simulink model "Supplementary_With_Disturbance"  (R2021a)
settings: Solver=ode4  StartTime=0.0  StopTime=30  FixedStep=0.01  RelTol=1e-3
PreLoadFcn:
  | A = [0	0.0203624760000000	0	0.253756485000000	0.195821163000000	-0.307147013000000	-0.0457249160000000	0	0.0294026210000000	0.282175234000000	0.145131294000000	-0.0517606740000000	0	-0.258258700000000	0.490455158000000	0.458982556000000	0.0397603470000000	0	0.458426005000000	-0.0485128840000000	0.0524025740000000	0.0287956120000000	0	0.0214875670000000	-0.232823046000000	-0.176253649000000	0.0308811180000000	0	-0.0210369990000000	-0.539800040000000	-0.0269942570000000
  | 0.0100000000000000	0.0199027140000000	0	0.254037792000000	0.198666794000000	-0.305673952000000	-0.0462416170000000	0	0.0268056150000000	0.287100361000000	0.149777099000000	-0.0521572690000000	0	-0.262654608000000	0.499529879000000	0.479520423000000	0.0400502210000000	0	0.458640154000000	-0.0508710880000000	0.0506368890000000	0.0290848310000000	0	0.0212556020000000	-0.238024528000000	-0.176409747000000	0.0238100370000000	0	-0.0279921310000000	-0.475815170000000	0.0106170450000000
  | 0.0200000000000000	0.0194376440000000	0	0.254292597000000	0.201563170000000	-0.304151471000000	-0.0467680610000000	0	0.0241495280000000	0.292165831000000	0.154721703000000	-0.0522047570000000	0	-0.266199871000000	0.505657970000000	0.494720708000000	0.0403420430000000	0	0.458851117000000	-0.0532733750000000	0.0488743790000000	0.0292718130000000	0	0.0209277250000000	-0.242339349000000	-0.176041308000000	0.0179082780000000	0	-0.0337221550000000	-0.422138031000000	0.0419436110000000
  | 0.0300000000000000	0.0189673530000000	0	0.254520783000000	0.204510111000000	-0.302579518000000	-0.0472857120000000	0	0.0214816170000000	0.297213520000000	0.159671513000000	-0.0513254030000000	0	-0.267382386000000	0.503879791000000	0.495241331000000	0.0406356570000000	0	0.459058709000000	-0.0557178750000000	0.0471160630000000	0.0294429970000000	0	0.0205811590000000	-0.246467289000000	-0.175570874000000	0.0163285640000000	0	-0.0355910120000000	-0.403449910000000	0.0521431170000000
  | 0.0400000000000000	0.0184919290000000	0	0.254722230000000	0.207507440000000	-0.300958041000000	-0.0477945690000000	0	0.0188018810000000	0.302243427000000	0.164626529000000	-0.0504460500000000	0	-0.268564901000000	0.502101612000000	0.495761953000000	0.0409309030000000	0	0.459262741000000	-0.0582027200000000	0.0453629610000000	0.0295983840000000	0	0.0202159040000000	-0.250408347000000	-0.174998446000000	0.0147488490000000	0	-0.0374598700000000	-0.384761789000000	0.0623426240000000
  | 0.0500000000000000	0.0180114610000000	0	0.254896820000000	0.210554980000000	-0.299286987000000	-0.0482946330000000	0	0.0161103190000000	0.307255552000000	0.169586752000000	-0.0495666960000000	0	-0.269747416000000	0.500323433000000	0.496282576000000	0.0412276250000000	0	0.459463027000000	-0.0607260420000000	0.0436160940000000	0.0297379740000000	0	0.0198319610000000	-0.254162524000000	-0.174324022000000	0.0131691350000000	0	-0.0393287270000000	-0.366073668000000	0.0725421300000000
  | 0.0600000000000000	0.0175260370000000	0	0.255044436000000	0.213652551000000	-0.297566306000000	-0.0487859030000000	0	0.0134069320000000	0.312249896000000	0.174552181000000	-0.0486873430000000	0	-0.270929931000000	0.498545254000000	0.496803199000000	0.0415256630000000	0	0.459659380000000	-0.0632859710000000	0.0418764810000000	0.0298617670000000	0	0.0194293300000000	-0.257729820000000	-0.173547603000000	0.0115894200000000	0	-0.0411975840000000	-0.347385547000000	0.0827416360000000
  | 0.0700000000000000	0.0170357430000000	0	0.255164959000000	0.216799977000000	-0.295795944000000	-0.0492683800000000	0	0.0106917200000000	0.317226458000000	0.179522816000000	-0.0478079890000000	0	-0.272112445000000	0.496767075000000	0.497323822000000	0.0418248600000000	0	0.459851613000000	-0.0658806380000000	0.0401451420000000	0.0299697620000000	0	0.0190080100000000	-0.261110235000000	-0.172669189000000	0.0100097060000000	0	-0.0430664410000000	-0.328697426000000	0.0929411430000000
  | 0.0800000000000000	0.0165406690000000	0	0.255258271000000	0.219997080000000	-0.293975849000000	-0.0497420630000000	0	0.00796468300000000	0.322185237000000	0.184498657000000	-0.0469286360000000	0	-0.273294960000000	0.494988895000000	0.497844444000000	0.0421250580000000	0	0.460039540000000	-0.0685081760000000	0.0384230970000000	0.0300619610000000	0	0.0185680010000000	-0.264303769000000	-0.171688780000000	0.00842999100000000	0	-0.0449352980000000	-0.310009305000000	0.103140649000000
  | 0.0900000000000000	0.0160409020000000	0	0.255324253000000	0.223243682000000	-0.292105971000000	-0.0502069520000000	0	0.00522582100000000	0.327126235000000	0.189479705000000	-0.0460492820000000	0	-0.274477475000000	0.493210716000000	0.498365067000000	0.0424260990000000	0	0.460222973000000	-0.0711667140000000	0.0367113660000000	0.0301383620000000	0	0.0181093040000000	-0.267310421000000	-0.170606376000000	0.00685027700000000	0	-0.0468041550000000	-0.291321184000000	0.113340155000000
  | 0.100000000000000	0.0155365300000000	0	0.255362787000000	0.226539605000000	-0.290186255000000	-0.0506630480000000	0	0.00247513400000000	0.332049452000000	0.194465959000000	-0.0451699290000000	0	-0.275659990000000	0.491432537000000	0.498885690000000	0.0427278250000000	0	0.460401726000000	-0.0738543840000000	0.0350109700000000	0.0301989660000000	0	0.0176319180000000	-0.270130193000000	-0.169421977000000	0.00527056200000000	0	-0.0486730120000000	-0.272633063000000	0.123539661000000
  | 0.110000000000000	0.0150276410000000	0	0.255373755000000	0.229884671000000	-0.288216651000000	-0.0511103510000000	0	-0.000287379000000000	0.336954886000000	0.199457419000000	-0.0442905750000000	0	-0.276842504000000	0.489654358000000	0.499406313000000	0.0430300780000000	0	0.460575612000000	-0.0765693180000000	0.0333229270000000	0.0302437740000000	0	0.0171358430000000	-0.272763083000000	-0.168135583000000	0.00369084800000000	0	-0.0505418690000000	-0.253944942000000	0.133739168000000
  | 0.120000000000000	0.0145143230000000	0	0.255357039000000	0.233278703000000	-0.286197107000000	-0.0515488600000000	0	-0.00306171600000000	0.341842539000000	0.204454085000000	-0.0434112220000000	0	-0.278025019000000	0.487876179000000	0.499926935000000	0.0433327010000000	0	0.460744443000000	-0.0793096460000000	0.0316482580000000	0.0302727830000000	0	0.0166210800000000	-0.275209091000000	-0.166747194000000	0.00211113400000000	0	-0.0524107270000000	-0.235256821000000	0.143938674000000
  | 0.130000000000000	0.0139966640000000	0	0.255312521000000	0.236721522000000	-0.284127570000000	-0.0519785750000000	0	-0.00584787900000000	0.346712410000000	0.209455957000000	-0.0425318690000000	0	-0.279207534000000	0.486098000000000	0.500447558000000	0.0436355340000000	0	0.460908033000000	-0.0820734990000000	0.0299879830000000	0.0302859960000000	0	0.0160876290000000	-0.277468219000000	-0.165256810000000	0.000531419000000000	0	-0.0542795840000000	-0.216568700000000	0.154138180000000
  | 0.140000000000000	0.0134747510000000	0	0.255240082000000	0.240212951000000	-0.282007988000000	-0.0523994970000000	0	-0.00864586700000000	0.351564499000000	0.214463036000000	-0.0416525150000000	0	-0.280390049000000	0.484319821000000	0.500968181000000	0.0439384210000000	0	0.461066196000000	-0.0848590100000000	0.0283431220000000	0.0302834120000000	0	0.0155354890000000	-0.279540465000000	-0.163664430000000	-0.00104829500000000	0	-0.0561484410000000	-0.197880579000000	0.164337687000000
  | 0.150000000000000	0.0129486740000000	0	0.255139604000000	0.243752812000000	-0.279838309000000	-0.0528116260000000	0	-0.0114556800000000	0.356398806000000	0.219475321000000	-0.0407731620000000	0	-0.281572564000000	0.482541642000000	0.501488804000000	0.0442412020000000	0	0.461218743000000	-0.0876643090000000	0.0267146940000000	0.0302650300000000	0	0.0149646600000000	-0.281425831000000	-0.161970056000000	-0.00262801000000000	0	-0.0580172980000000	-0.179192458000000	0.174537193000000
  | 0.160000000000000	0.0124185190000000	0	0.255010968000000	0.247340927000000	-0.277618481000000	-0.0532149610000000	0	-0.0142773180000000	0.361215332000000	0.224492812000000	-0.0398938080000000	0	-0.282755078000000	0.480763463000000	0.502009426000000	0.0445437210000000	0	0.461365489000000	-0.0904875270000000	0.0251037210000000	0.0302308520000000	0	0.0143751430000000	-0.283124315000000	-0.160173686000000	-0.00420772400000000	0	-0.0598861550000000	-0.160504337000000	0.184736699000000
  | 0.170000000000000	0.0118843750000000	0	0.254854057000000	0.250977119000000	-0.275348453000000	-0.0536095020000000	0	-0.0171107810000000	0.366014075000000	0.229515510000000	-0.0390144550000000	0	-0.283937593000000	0.478985283000000	0.502530049000000	0.0448458190000000	0	0.461506246000000	-0.0933267950000000	0.0235112210000000	0.0301808760000000	0	0.0137669370000000	-0.284635917000000	-0.158275322000000	-0.00578743900000000	0	-0.0617550120000000	-0.141816216000000	0.194936206000000
  | 0.180000000000000	0.0113463290000000	0	0.254668753000000	0.254661209000000	-0.273028171000000	-0.0539952500000000	0	-0.0199560700000000	0.370795037000000	0.234543413000000	-0.0381351010000000	0	-0.285120108000000	0.477207104000000	0.503050672000000	0.0451473390000000	0	0.461640827000000	-0.0961802450000000	0.0219382140000000	0.0301151030000000	0	0.0131400430000000	-0.285960639000000	-0.156274962000000	-0.00736715300000000	0	-0.0636238690000000	-0.123128095000000	0.205135712000000
  | 0.190000000000000	0.0108044700000000	0	0.254454936000000	0.258393019000000	-0.270657584000000	-0.0543722040000000	0	-0.0228131840000000	0.375558218000000	0.239576523000000	-0.0372471780000000	0	-0.286274649000000	0.475350099000000	0.503402990000000	0.0454481210000000	0	0.461769047000000	-0.0990460080000000	0.0203857210000000	0.0300335330000000	0	0.0124944600000000	-0.287098479000000	-0.154172608000000	-0.00891109700000000	0	-0.0654632260000000	-0.104750233000000	0.215162082000000
  | 0.200000000000000	0.0102588850000000	0	0.254212489000000	0.262172373000000	-0.268236641000000	-0.0547401930000000	0	-0.0256815630000000	0.380302039000000	0.244611473000000	-0.0363078340000000	0	-0.287261343000000	0.473020134000000	0.502745482000000	0.0457480090000000	0	0.461890717000000	-0.101922215000000	0.0188547620000000	0.0299368810000000	0	0.0118307780000000	-0.288055644000000	-0.151971721000000	-0.0102404190000000	0	-0.0671255790000000	-0.0882339300000000	0.224149638000000
  | 0.210000000000000	0.00970966600000000	0	0.253941305000000	0.265999060000000	-0.265765355000000	-0.0550983610000000	0	-0.0285584100000000	0.385018620000000	0.249631433000000	-0.0352827890000000	0	-0.287968296000000	0.469901904000000	0.500404928000000	0.0460468590000000	0	0.462005662000000	-0.104807121000000	0.0173462870000000	0.0298287240000000	0	0.0111519480000000	-0.288863158000000	-0.149689615000000	-0.0112120360000000	0	-0.0684929260000000	-0.0748202250000000	0.231405835000000
  | 0.220000000000000	0.00915691800000000	0	0.253641321000000	0.269872745000000	-0.263244012000000	-0.0554458490000000	0	-0.0314409290000000	0.389700077000000	0.254619572000000	-0.0342063240000000	0	-0.288507402000000	0.466310715000000	0.497054548000000	0.0463445840000000	0	0.462113756000000	-0.107699478000000	0.0158609700000000	0.0297126400000000	0	0.0104609200000000	-0.289552048000000	-0.147343604000000	-0.0119690300000000	0	-0.0696832690000000	-0.0632680770000000	0.237623216000000
  | 0.230000000000000	0.00860074900000000	0	0.253312486000000	0.273793062000000	-0.260672964000000	-0.0557824870000000	0	-0.0343285590000000	0.394344834000000	0.259572524000000	-0.0331212890000000	0	-0.289018535000000	0.462640699000000	0.493535862000000	0.0466411120000000	0	0.462214881000000	-0.110598162000000	0.0143994150000000	0.0295893440000000	0	0.00975828300000000	-0.290128519000000	-0.144937151000000	-0.0126902540000000	0	-0.0708441120000000	-0.0520261900000000	0.243667462000000
  | 0.240000000000000	0.00804126800000000	0	0.252954750000000	0.277759642000000	-0.258052562000000	-0.0561082750000000	0	-0.0372213000000000	0.398952891000000	0.264490289000000	-0.0320362530000000	0	-0.289529667000000	0.458970684000000	0.490017177000000	0.0469363710000000	0	0.462308921000000	-0.113502048000000	0.0129622270000000	0.0294588350000000	0	0.00904403700000000	-0.290592572000000	-0.142470255000000	-0.0134114780000000	0	-0.0720049540000000	-0.0407843020000000	0.249711708000000
  | 0.250000000000000	0.00747858300000000	0	0.252568060000000	0.281772120000000	-0.255383158000000	-0.0564232120000000	0	-0.0401191520000000	0.403524248000000	0.269372867000000	-0.0309512180000000	0	-0.290040799000000	0.455300668000000	0.486498492000000	0.0472302890000000	0	0.462395761000000	-0.116410013000000	0.0115500100000000	0.0293211140000000	0	0.00831818400000000	-0.290944205000000	-0.139942916000000	-0.0141327030000000	0	-0.0731657970000000	-0.0295424150000000	0.255755954000000
  | 0.260000000000000	0.00691280400000000	0	0.252152367000000	0.285830127000000	-0.252665104000000	-0.0567272990000000	0	-0.0430221160000000	0.408058905000000	0.274220259000000	-0.0298661830000000	0	-0.290551932000000	0.451630652000000	0.482979807000000	0.0475227930000000	0	0.462475285000000	-0.119320932000000	0.0101633690000000	0.0291761810000000	0	0.00758072100000000	-0.291183420000000	-0.137355136000000	-0.0148539270000000	0	-0.0743266400000000	-0.0183005270000000	0.261800200000000
  | 0.270000000000000	0.00634403700000000	0	0.251707618000000	0.289933298000000	-0.249898753000000	-0.0570205360000000	0	-0.0459301910000000	0.412556861000000	0.279032463000000	-0.0287811480000000	0	-0.291063064000000	0.447960637000000	0.479461122000000	0.0478138120000000	0	0.462547376000000	-0.122233682000000	0.00880290700000000	0.0290240360000000	0	0.00683165100000000	-0.291310216000000	-0.134706912000000	-0.0155751510000000	0	-0.0754874820000000	-0.00705864000000000	0.267844446000000
  | 0.280000000000000	0.00577239300000000	0	0.251233763000000	0.294081264000000	-0.247084455000000	-0.0573029220000000	0	-0.0488433770000000	0.417018117000000	0.283809481000000	-0.0276961130000000	0	-0.291574197000000	0.444290621000000	0.475942437000000	0.0481032740000000	0	0.462611918000000	-0.125147137000000	0.00746923000000000	0.0288646780000000	0	0.00607097200000000	-0.291324593000000	-0.131998247000000	-0.0162963750000000	0	-0.0766483250000000	0.00418324800000000	0.273888692000000
  | 0.290000000000000	0.00519797900000000	0	0.250730750000000	0.298273660000000	-0.244222563000000	-0.0575744580000000	0	-0.0517616740000000	0.421442674000000	0.288551312000000	-0.0266059110000000	0	-0.292060919000000	0.440564738000000	0.472282299000000	0.0483911060000000	0	0.462668795000000	-0.128060173000000	0.00616294200000000	0.0286981080000000	0	0.00529868400000000	-0.291226551000000	-0.129229138000000	-0.0170007460000000	0	-0.0777982440000000	0.0152544010000000	0.279849410000000
  | 0.300000000000000	0.00462090400000000	0	0.250198529000000	0.302510118000000	-0.241313429000000	-0.0578350400000000	0	-0.0546845950000000	0.425829412000000	0.293255127000000	-0.0254847100000000	0	-0.292401181000000	0.436503650000000	0.467773438000000	0.0486772360000000	0	0.462717892000000	-0.130971668000000	0.00488464800000000	0.0285246630000000	0	0.00451500700000000	-0.291019505000000	-0.126401258000000	-0.0176040010000000	0	-0.0788826220000000	0.0253011480000000	0.285308954000000
  | 0.310000000000000	0.00404127800000000	0	0.249637058000000	0.306790248000000	-0.238357460000000	-0.0580841520000000	0	-0.0576096980000000	0.430172747000000	0.297906781000000	-0.0243118440000000	0	-0.292497344000000	0.431883887000000	0.461850039000000	0.0489615990000000	0	0.462759095000000	-0.133880564000000	0.00363491700000000	0.0283460280000000	0	0.00372103200000000	-0.290720528000000	-0.123522959000000	-0.0180387280000000	0	-0.0798577640000000	0.0336405530000000	0.289933211000000
  | 0.320000000000000	0.00345922100000000	0	0.249046335000000	0.311113573000000	-0.235355293000000	-0.0583212770000000	0	-0.0605345420000000	0.434467090000000	0.302492128000000	-0.0231079780000000	0	-0.292447047000000	0.426928918000000	0.455077919000000	0.0492441560000000	0	0.462792312000000	-0.136786078000000	0.00241418800000000	0.0281638890000000	0	0.00291785200000000	-0.290346694000000	-0.120602594000000	-0.0183723380000000	0	-0.0807673640000000	0.0409555520000000	0.294056294000000
  | 0.330000000000000	0.00287485300000000	0	0.248426368000000	0.315479590000000	-0.232307618000000	-0.0585463120000000	0	-0.0634586390000000	0.438711325000000	0.307008339000000	-0.0218989460000000	0	-0.292372340000000	0.421918082000000	0.448164344000000	0.0495248770000000	0	0.462817452000000	-0.139687497000000	0.00122286500000000	0.0279785810000000	0	0.00210568500000000	-0.289901417000000	-0.117641834000000	-0.0186890960000000	0	-0.0816660410000000	0.0480998160000000	0.298095849000000
  | 0.340000000000000	0.00228829400000000	0	0.247777163000000	0.319887799000000	-0.229215126000000	-0.0587592560000000	0	-0.0663819890000000	0.442905452000000	0.311455415000000	-0.0206899140000000	0	-0.292297633000000	0.416907247000000	0.441250770000000	0.0498037280000000	0	0.462834426000000	-0.142584107000000	6.13517000000000e-05	0.0277901070000000	0	0.00128453100000000	-0.289384698000000	-0.114640677000000	-0.0190058540000000	0	-0.0825647180000000	0.0552440800000000	0.302135404000000
  | 0.350000000000000	0.00169966700000000	0	0.247098728000000	0.324337699000000	-0.226078510000000	-0.0589601100000000	0	-0.0693045920000000	0.447049470000000	0.315833355000000	-0.0194808810000000	0	-0.292222926000000	0.411896411000000	0.434337196000000	0.0500806790000000	0	0.462843143000000	-0.145475191000000	-0.00106994800000000	0.0275984640000000	0	0.000454390000000000	-0.288796535000000	-0.111599125000000	-0.0193226120000000	0	-0.0834633940000000	0.0623883450000000	0.306174959000000
  | 0.360000000000000	0.00110909200000000	0	0.246391071000000	0.328828789000000	-0.222898459000000	-0.0591488740000000	0	-0.0722264470000000	0.451143380000000	0.320142159000000	-0.0182718490000000	0	-0.292148219000000	0.406885575000000	0.427423621000000	0.0503556970000000	0	0.462843514000000	-0.148360037000000	-0.00217063100000000	0.0274036540000000	0	-0.000384737000000000	-0.288136931000000	-0.108517178000000	-0.0196393690000000	0	-0.0843620710000000	0.0695326090000000	0.310214514000000
  | 0.370000000000000	0.000516690000000000	0	0.245654199000000	0.333360567000000	-0.219675666000000	-0.0593255470000000	0	-0.0751475560000000	0.455187181000000	0.324381827000000	-0.0170628170000000	0	-0.292073512000000	0.401874739000000	0.420510047000000	0.0506287520000000	0	0.462835448000000	-0.151237930000000	-0.00324029200000000	0.0272056770000000	0	-0.00123285100000000	-0.287405883000000	-0.105394835000000	-0.0199561270000000	0	-0.0852607480000000	0.0766768730000000	0.314254069000000
  | 0.380000000000000	-7.74187000000000e-05	0	0.244888120000000	0.337932532000000	-0.216410823000000	-0.0594901300000000	0	-0.0780679180000000	0.459180875000000	0.328552360000000	-0.0158537850000000	0	-0.291998805000000	0.396863903000000	0.413596473000000	0.0508998110000000	0	0.462818857000000	-0.154108155000000	-0.00427852800000000	0.0270045320000000	0	-0.00208995200000000	-0.286603393000000	-0.102232097000000	-0.0202728850000000	0	-0.0861594250000000	0.0838211380000000	0.318293624000000
  | 0.390000000000000	-0.000673113000000000	0	0.244092840000000	0.342544184000000	-0.213104619000000	-0.0596426230000000	0	-0.0809875320000000	0.463124459000000	0.332653756000000	-0.0146402710000000	0	-0.291897151000000	0.391796177000000	0.406533095000000	0.0511688430000000	0	0.462793649000000	-0.156969998000000	-0.00528493400000000	0.0268002190000000	0	-0.00295604000000000	-0.285729461000000	-0.0990289630000000	-0.0205761090000000	0	-0.0870513460000000	0.0908152870000000	0.322260174000000
  | 0.400000000000000	-0.00127027100000000	0	0.243268369000000	0.347195021000000	-0.209757747000000	-0.0597829360000000	0	-0.0839058610000000	0.467016798000000	0.336683021000000	-0.0133998700000000	0	-0.291633811000000	0.386387108000000	0.398570900000000	0.0514358150000000	0	0.462759736000000	-0.159822744000000	-0.00625910700000000	0.0265930100000000	0	-0.00383097900000000	-0.284787087000000	-0.0957868930000000	-0.0207981340000000	0	-0.0879027380000000	0.0969087460000000	0.325788692000000
  | 0.410000000000000	-0.00186877100000000	0	0.242414723000000	0.351884520000000	-0.206370959000000	-0.0599106200000000	0	-0.0868202080000000	0.470852202000000	0.340625174000000	-0.0121146550000000	0	-0.291100997000000	0.380409136000000	0.389110674000000	0.0517007030000000	0	0.462717030000000	-0.162665740000000	-0.00720067200000000	0.0263842570000000	0	-0.00471409400000000	-0.283791286000000	-0.0925131890000000	-0.0208848250000000	0	-0.0886865810000000	0.101501054000000	0.328587159000000
  | 0.420000000000000	-0.00246848400000000	0	0.241531965000000	0.356612065000000	-0.202945244000000	-0.0600252290000000	0	-0.0897278810000000	0.474624981000000	0.344465235000000	-0.0108025530000000	0	-0.290406497000000	0.374089821000000	0.378751630000000	0.0519635000000000	0	0.462665454000000	-0.165498570000000	-0.00810937100000000	0.0261753130000000	0	-0.00560471100000000	-0.282757066000000	-0.0892151500000000	-0.0208903160000000	0	-0.0894298930000000	0.105192671000000	0.330947593000000
  | 0.430000000000000	-0.00306927600000000	0	0.240620166000000	0.361377020000000	-0.199481654000000	-0.0601266710000000	0	-0.0926283380000000	0.478333998000000	0.348200207000000	-0.00948596900000000	0	-0.289685050000000	0.367713616000000	0.368242783000000	0.0522242090000000	0	0.462604935000000	-0.168320881000000	-0.00898497500000000	0.0259664500000000	0	-0.00650269200000000	-0.281687432000000	-0.0858942370000000	-0.0208822740000000	0	-0.0901664510000000	0.108734174000000	0.333235023000000
  | 0.440000000000000	-0.00367101700000000	0	0.239679398000000	0.366178745000000	-0.195981240000000	-0.0602149480000000	0	-0.0955215820000000	0.481979253000000	0.351830091000000	-0.00816938500000000	0	-0.288963603000000	0.361337411000000	0.357733935000000	0.0524828290000000	0	0.462535400000000	-0.171132319000000	-0.00982725500000000	0.0257576680000000	0	-0.00740804000000000	-0.280582383000000	-0.0825504500000000	-0.0208742330000000	0	-0.0909030080000000	0.112275676000000	0.335522453000000
  | 0.450000000000000	-0.00427357500000000	0	0.238709734000000	0.371016605000000	-0.192445052000000	-0.0602900590000000	0	-0.0984076100000000	0.485560746000000	0.355354886000000	-0.00685280100000000	0	-0.288242156000000	0.354961205000000	0.347225088000000	0.0527393620000000	0	0.462456775000000	-0.173932529000000	-0.0106359840000000	0.0255489660000000	0	-0.00832075200000000	-0.279441919000000	-0.0791837880000000	-0.0208661910000000	0	-0.0916395660000000	0.115817178000000	0.337809882000000
  | 0.460000000000000	-0.00487681800000000	0	0.237711246000000	0.375889960000000	-0.188874142000000	-0.0603520040000000	0	-0.101286425000000	0.489078477000000	0.358774592000000	-0.00553621800000000	0	-0.287520709000000	0.348585000000000	0.336716241000000	0.0529938090000000	0	0.462368985000000	-0.176721157000000	-0.0114109310000000	0.0253403440000000	0	-0.00924083100000000	-0.278266039000000	-0.0757942520000000	-0.0208581490000000	0	-0.0923761230000000	0.119358681000000	0.340097312000000
  | 0.470000000000000	-0.00548061500000000	0	0.236684006000000	0.380798174000000	-0.185269560000000	-0.0604007830000000	0	-0.104158025000000	0.492532446000000	0.362089211000000	-0.00421963400000000	0	-0.286799262000000	0.342208795000000	0.326207394000000	0.0532461690000000	0	0.462271958000000	-0.179497849000000	-0.0121518690000000	0.0251318030000000	0	-0.0101682750000000	-0.277054745000000	-0.0723818420000000	-0.0208501070000000	0	-0.0931126810000000	0.122900183000000	0.342384742000000
  | 0.480000000000000	-0.00608483400000000	0	0.235628085000000	0.385740609000000	-0.181632358000000	-0.0604363970000000	0	-0.107022410000000	0.495922653000000	0.365298740000000	-0.00290305000000000	0	-0.286077815000000	0.335832590000000	0.315698547000000	0.0534964450000000	0	0.462165620000000	-0.182262252000000	-0.0128585680000000	0.0249233420000000	0	-0.0111030850000000	-0.275808036000000	-0.0689465570000000	-0.0208420650000000	0	-0.0938492380000000	0.126441685000000	0.344672171000000
  | 0.490000000000000	-0.00668934300000000	0	0.234543557000000	0.390716627000000	-0.177963586000000	-0.0604588440000000	0	-0.109879581000000	0.499249098000000	0.368403182000000	-0.00158392300000000	0	-0.285330855000000	0.329408201000000	0.305061362000000	0.0537446360000000	0	0.462049896000000	-0.185014010000000	-0.0135308000000000	0.0247149610000000	0	-0.0120452600000000	-0.274525911000000	-0.0654883980000000	-0.0208268820000000	0	-0.0945850800000000	0.129883526000000	0.346908955000000
  | 0.500000000000000	-0.00729401100000000	0	0.233430494000000	0.395725591000000	-0.174264294000000	-0.0604680750000000	0	-0.112729027000000	0.502510817000000	0.371399968000000	-0.000249539000000000	0	-0.284430817000000	0.322694708000000	0.293654148000000	0.0539907440000000	0	0.461924715000000	-0.187752770000000	-0.0141683360000000	0.0245068040000000	0	-0.0129947860000000	-0.273210365000000	-0.0620083780000000	-0.0207688540000000	0	-0.0953166300000000	0.132727399000000	0.348841864000000
  | 0.510000000000000	-0.00789870400000000	0	0.232288977000000	0.400766844000000	-0.170535586000000	-0.0604638350000000	0	-0.115568197000000	0.505702992000000	0.374276264000000	0.00111027500000000	0	-0.283275650000000	0.315499377000000	0.280963555000000	0.0542347720000000	0	0.461790001000000	-0.190478217000000	-0.0147709670000000	0.0242995840000000	0	-0.0139515920000000	-0.271871363000000	-0.0585115610000000	-0.0206394170000000	0	-0.0960410250000000	0.134574657000000	0.350268315000000
  | 0.520000000000000	-0.00850328700000000	0	0.231119130000000	0.405839651000000	-0.166778769000000	-0.0604458700000000	0	-0.118394540000000	0.508820805000000	0.377019239000000	0.00248534600000000	0	-0.281967406000000	0.308014942000000	0.267502933000000	0.0544767360000000	0	0.461645683000000	-0.193190197000000	-0.0153385670000000	0.0240940160000000	0	-0.0149156070000000	-0.270518872000000	-0.0550030120000000	-0.0204671340000000	0	-0.0967611270000000	0.135823947000000	0.351390891000000
  | 0.530000000000000	-0.00910762200000000	0	0.229921086000000	0.410943260000000	-0.162995201000000	-0.0604141280000000	0	-0.121207545000000	0.511863291000000	0.379626323000000	0.00386296000000000	0	-0.280633649000000	0.300482323000000	0.253913973000000	0.0547166530000000	0	0.461491689000000	-0.195888595000000	-0.0158710280000000	0.0238902420000000	0	-0.0158868150000000	-0.269154884000000	-0.0514837430000000	-0.0202877100000000	0	-0.0974805150000000	0.136973576000000	0.352462821000000
  | 0.540000000000000	-0.00971157000000000	0	0.228694979000000	0.416076917000000	-0.159186243000000	-0.0603686100000000	0	-0.124007213000000	0.514830451000000	0.382097518000000	0.00524057500000000	0	-0.279299892000000	0.292949704000000	0.240325013000000	0.0549545410000000	0	0.461327946000000	-0.198573295000000	-0.0163682420000000	0.0236882620000000	0	-0.0168652170000000	-0.267779401000000	-0.0479537550000000	-0.0201082860000000	0	-0.0981999020000000	0.138123204000000	0.353534751000000
  | 0.550000000000000	-0.0103149940000000	0	0.227440942000000	0.421239869000000	-0.155353251000000	-0.0603093170000000	0	-0.126793543000000	0.517722285000000	0.384432823000000	0.00661818900000000	0	-0.277966135000000	0.285417085000000	0.226736054000000	0.0551904180000000	0	0.461154384000000	-0.201244183000000	-0.0168301030000000	0.0234880760000000	0	-0.0178508130000000	-0.266392420000000	-0.0444130480000000	-0.0199288620000000	0	-0.0989192890000000	0.139272833000000	0.354606681000000
  | 0.560000000000000	-0.0109177560000000	0	0.226159108000000	0.426431363000000	-0.151497586000000	-0.0602362470000000	0	-0.129566536000000	0.520538793000000	0.386632239000000	0.00799580400000000	0	-0.276632378000000	0.277884466000000	0.213147094000000	0.0554243020000000	0	0.460970930000000	-0.203901143000000	-0.0172565030000000	0.0232896840000000	0	-0.0188436030000000	-0.264993944000000	-0.0408616220000000	-0.0197494390000000	0	-0.0996386760000000	0.140422461000000	0.355678611000000
  | 0.570000000000000	-0.0115197190000000	0	0.224849611000000	0.431650645000000	-0.147620606000000	-0.0601494010000000	0	-0.132326191000000	0.523279974000000	0.388695765000000	0.00937341800000000	0	-0.275298621000000	0.270351848000000	0.199558134000000	0.0556562110000000	0	0.460777512000000	-0.206544062000000	-0.0176473350000000	0.0230930870000000	0	-0.0198435860000000	-0.263583971000000	-0.0372994760000000	-0.0195700150000000	0	-0.100358063000000	0.141572090000000	0.356750541000000
  | 0.580000000000000	-0.0121207440000000	0	0.223512584000000	0.436896962000000	-0.143723671000000	-0.0600487780000000	0	-0.135072508000000	0.525945830000000	0.390623402000000	0.0107510320000000	0	-0.273964863000000	0.262819229000000	0.185969174000000	0.0558861640000000	0	0.460574058000000	-0.209172823000000	-0.0180024920000000	0.0228982840000000	0	-0.0208507640000000	-0.262162502000000	-0.0337266110000000	-0.0193905910000000	0	-0.101077450000000	0.142721718000000	0.357822471000000
  | 0.590000000000000	-0.0127206950000000	0	0.222148161000000	0.442169561000000	-0.139808138000000	-0.0599343800000000	0	-0.137805488000000	0.528536359000000	0.392415149000000	0.0121290720000000	0	-0.272608235000000	0.255247885000000	0.172286638000000	0.0561141770000000	0	0.460360497000000	-0.211787312000000	-0.0183218670000000	0.0227052750000000	0	-0.0218651350000000	-0.260729537000000	-0.0301430260000000	-0.0192084990000000	0	-0.101799218000000	0.143810206000000	0.358853518000000
  | ... (+5941 lines)
StopFcn:
  | clc
  | close all
  | 
  | T = Time.Data(:);
  | 
  | 
  | LeftThighF = LThighF.Data(:,:);
  | LeftThighT = LThighT.Data(:,:);
  | LeftThighS = LThighS.Data(:,:);
  | LeftKnee   = LKnee.Data(:,:);
  | LeftAnkle  = LAnkle.Data(:,:);
  | 
  | RightThighF = RThighF.Data(:,:);
  | RightThighT = RThighT.Data(:,:);
  | RightThighS = RThighS.Data(:,:);
  | RightKnee   = RKnee.Data(:,:);
  | RightAnkle  = RAnkle.Data(:,:);
  | 
  | 
  | LeftThighFtorque = LThighFtorque.Data(:);
  | LeftThighTtorque = LThighTtorque.Data(:);
  | LeftThighStorque = LThighStorque.Data(:);
  | LeftKneetorque   = LKneetorque.Data(:);
  | LeftAnkletorque  = LAnkletorque.Data(:);
  | 
  | RightThighFtorque = RThighFtorque.Data(:);
  | RightThighTtorque = RThighTtorque.Data(:);
  | RightThighStorque = RThighStorque.Data(:);
  | RightKneetorque   = RKneetorque.Data(:);
  | RightAnkletorque  = RAnkletorque.Data(:);
  | 
  | 
  | figure
  | subplot(4,2,2)
  | plot(T,RightThighF(:,1),'g',T,RightThighF(:,2),'b',T,RightThighF(:,3),'--m' ,'LineWidth',3)
  | legend({'\theta_{Ref}','\theta_{Simscape}','\theta_{Simulink}'}, 'Location','northeast', 'FontSize',10,'FontName', 'Times New Roman', 'FontWeight', 'bold')
  | xlabel('Time (Sec)', 'FontSize',10,'FontName', 'Times New Roman', 'FontWeight', 'bold' )
  | ylabel('Position (Degree)', 'FontSize',10,'FontName', 'Times New Roman', 'FontWeight', 'bold' )
  | title('Right Frontal Hip Position', 'FontSize',10,'FontName', 'Times New Roman' , 'FontWeight', 'bold')
  | ax = gca;
  | ax.FontSize = 10;
  | ax.FontName = 'Times New Roman';
  | ax.FontWeight = 'bold';
  | grid on
  | 
  | 
  | 
  | subplot(4,2,4)
  | plot(T,RightThighS(:,1),'g',T,RightThighS(:,2),'b',T,RightThighS(:,3),'--m' ,'LineWidth',3)
  | legend({'\theta_{Ref}','\theta_{Simscape}','\theta_{Simulink}'}, 'Location','northeast', 'FontSize',10,'FontName', 'Times New Roman', 'FontWeight', 'bold')
  | xlabel('Time (Sec)', 'FontSize',10,'FontName', 'Times New Roman', 'FontWeight', 'bold' )
  | ylabel('Position (Degree)', 'FontSize',10,'FontName', 'Times New Roman', 'FontWeight', 'bold' )
  | title('Right Saggital Hip Position', 'FontSize',10,'FontName', 'Times New Roman' , 'FontWeight', 'bold')
  | ax = gca;
  | ax.FontSize = 10;
  | ax.FontName = 'Times New Roman';
  | ax.FontWeight = 'bold';
  | grid on
  | 
  | 
  | ... (+135 lines)
undefined symbols (not defined in the file): X, Y, Z
libraries: sm_lib x34, nesl_utility x26, simulink x1
(part 23 of 51)

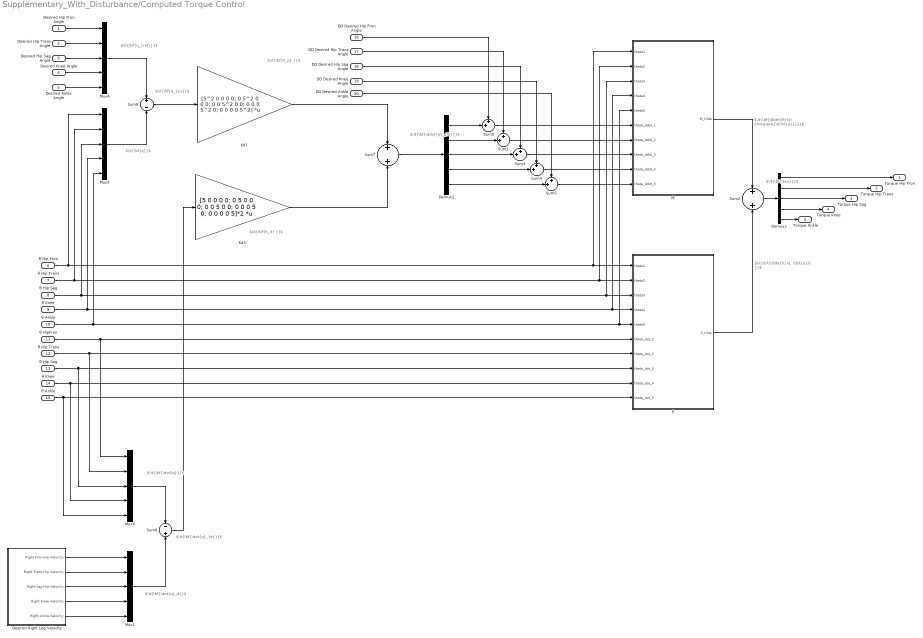
== system Supplementary_With_Disturbance/Computed Torque Control ==
  note: $\it{\bf{\tilde{M}(q) \thinspace{\ddot{q}}}}}$
  note: $\it{\bf{q}}$
  note: $\it{\bf{q_{ref}}}$
  note: $\it{\bf{\tilde{h}(q, \dot{q})} }}$
  note: $\it{\bf{\tau}}}$
  note: $\it{\bf{q_{e}}}$
  note: $\it{\bf{K_p} }}$
  note: $\it{\bf{\dot{q}}}$
  note: $\it{\bf{\dot{q}_d}}$
  note: $\it{\bf{K_d} }}$
  note: $\it{\bf{\dot{q}_{e}}}$
  note: $\it{\bf{\ddot{q}_{fb}}}$
  Desired Hip Fron Angle : Inport
  Desired Hip Trans Angle : Inport  Port=2
  Desired Hip Sag Angle : Inport  Port=3
  Desired Knee Angle : Inport  Port=4
  Desired Ankle Angle : Inport  Port=5
  θ Hip Fron : Inport  Port=6
  θ Hip Trans : Inport  Port=7
  θ Hip Sag : Inport  Port=8
  θ Knee : Inport  Port=9
  θ Ankle : Inport  Port=10
  θ́ HipFron : Inport  Port=11
  θ́ Hip Trans : Inport  Port=12
  θ́ Hip Sag : Inport  Port=13
  θ́ Knee : Inport  Port=14
  θ́ Ankle : Inport  Port=15
  DD Desired Hip Fron Angle : Inport  Port=16
  DD Desired Hip Trans Angle : Inport  Port=17
  DD Desired Hip Sag Angle : Inport  Port=18
  DD Desired Knee Angle : Inport  Port=19
  DD Desired Ankle Angle : Inport  Port=20
  " h͂" : MATLAB Function  TreatAsAtomicUnit=on
  Demux1 : Demux  Outputs=5
  Demux2 : Demux  Outputs=5
  Desired Right Leg Velocity : Subsystem
      mask Display:
      | port_label('output',1,'\theta\prime_d_{ Hip Frontal}','texmode','on');
      | port_label('output',2,'\theta\prime_d_{ Hip Trans}','texmode','on');
      | port_label('output',3,'\theta\prime_d_{ Hip Saggital}','texmode','on');
      | port_label('output',4,'\theta\prime_d_{ Knee}','texmode','on');
      | port_label('output',5,'\theta\prime_d_{ Ankle}','texmode','on');
  Kd1 : Gain  Gain="[5^2  0  0  0  0; 0  5^2  0  0  0; 0  0  5^2  0  0; 0  0  0  5^2  0; 0  0  0  0  5^2]"  Multiplication=Matrix(K*u) (u vector)
  Kd3 : Gain  Gain="[5  0  0  0  0; 0  5  0  0  0; 0  0  5  0  0; 0  0  0  5  0; 0  0  0  0  5]*2"  Multiplication=Matrix(K*u) (u vector)
  Mux{1,4..6} (4 alike) : Mux  Inputs=5
  M͂ : MATLAB Function  TreatAsAtomicUnit=on
  Sum{1,3..5,9} (5 alike) : Sum  Inputs=++|
  Sum2 : Sum
  Sum6 : Sum  Inputs=+-
  Sum7 : Sum
  Sum8 : Sum  Inputs=-+
  Torque Hip Fron : Outport
  Torque Hip Trans : Outport  Port=2
  Torque Hip Sag : Outport  Port=3
  Torque Knee : Outport  Port=4
  Torque Ankle : Outport  Port=5
  wires:
  θ́ Hip Sag/1 -> " h͂"/8(theta_dot_3), Mux6/3
  θ́ Knee/1 -> " h͂"/9(theta_dot_4), Mux6/4
  θ́ Ankle/1 -> " h͂"/10(theta_dot_5), Mux6/5
  θ Hip Sag/1 -> " h͂"/3(theta3), M͂/3(theta3), Mux5/3
  θ Knee/1 -> Mux5/4, " h͂"/4(theta4), M͂/4(theta4)
  θ Ankle/1 -> Mux5/5, M͂/5(theta5), " h͂"/5(theta5)
  " h͂"/1(h_tilda) -> Sum2/2
  M͂/1(M_tilda) -> Sum2/1
  Sum2/1 -> Demux1/1
  DD Desired Hip Sag Angle/1 -> Sum3/1
  DD Desired Knee Angle/1 -> Sum4/1
  DD Desired Ankle Angle/1 -> Sum5/1
  Mux4/1 -> Sum6/1
  Mux5/1 -> Sum6/2
  Sum6/1 -> Kd1/1
  Kd1/1 -> Sum7/1
  Sum7/1 -> Demux2/1
  Mux1/1 -> Sum8/2
  Mux6/1 -> Sum8/1
  Sum8/1 -> Kd3/1
  Sum4/1 -> M͂/9(theta_ddot_4)
  Demux1/5 -> Torque Ankle/1
  Demux1/4 -> Torque Knee/1
  Demux1/3 -> Torque Hip Sag/1
  Demux1/1 -> Torque Hip Fron/1
  Demux1/2 -> Torque Hip Trans/1
  Desired Ankle Angle/1 -> Mux4/5
  Desired Knee Angle/1 -> Mux4/4
  Desired Hip Sag Angle/1 -> Mux4/3
  Desired Hip Fron Angle/1 -> Mux4/1
  Desired Hip Trans Angle/1 -> Mux4/2
  θ Hip Fron/1 -> M͂/1(theta1), " h͂"/1(theta1), Mux5/1
  θ Hip Trans/1 -> " h͂"/2(theta2), M͂/2(theta2), Mux5/2
  θ́ Hip Trans/1 -> " h͂"/7(theta_dot_2), Mux6/2
  θ́ HipFron/1 -> Mux6/1, " h͂"/6(theta_dot_1)
  Desired Right Leg Velocity/1(Right Fron Hip Velocity) -> Mux1/1
  Desired Right Leg Velocity/2(Right Trans Hip Velocity) -> Mux1/2
  Desired Right Leg Velocity/3(Right Sag Hip Velocity) -> Mux1/3
  Desired Right Leg Velocity/4(Right Knee Velocity) -> Mux1/4
  Desired Right Leg Velocity/5(Right Ankle Velocity) -> Mux1/5
  Demux2/5 -> Sum5/2
  Demux2/4 -> Sum4/2
  Sum5/1 -> M͂/10(theta_ddot_5)
  Demux2/3 -> Sum3/2
  Sum3/1 -> M͂/8(theta_ddot_3)
  Demux2/2 -> Sum1/2
  Sum1/1 -> M͂/7(theta_ddot_2)
  Demux2/1 -> Sum9/2
  Sum9/1 -> M͂/6(theta_ddot_1)
  DD Desired Hip Fron Angle/1 -> Sum9/1
  DD Desired Hip Trans Angle/1 -> Sum1/1
  Kd3/1 -> Sum7/2

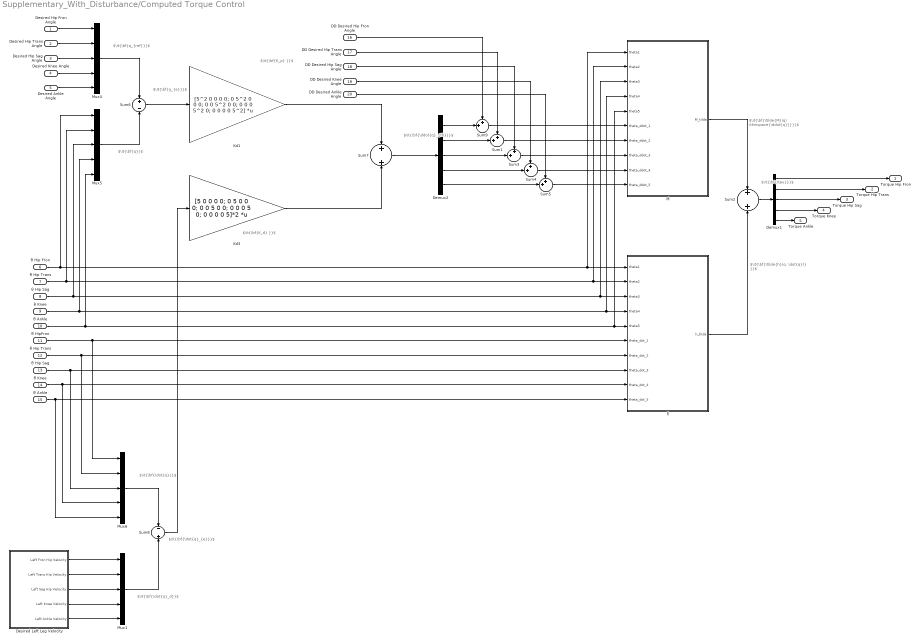
== system Supplementary_With_Disturbance/Computed Torque Control  ==
  note: $\it{\bf{\tilde{M}(q) \thinspace{\ddot{q}}}}}$
  note: $\it{\bf{q}}$
  note: $\it{\bf{q_{ref}}}$
  note: $\it{\bf{\tilde{h}(q, \dot{q})} }}$
  note: $\it{\bf{\tau}}}$
  note: $\it{\bf{q_{e}}}$
  note: $\it{\bf{K_p} }}$
  note: $\it{\bf{\dot{q}}}$
  note: $\it{\bf{\dot{q}_d}}$
  note: $\it{\bf{K_d} }}$
  note: $\it{\bf{\dot{q}_{e}}}$
  note: $\it{\bf{\ddot{q}_{fb}}}$
  Desired Hip Fron Angle : Inport
  Desired Hip Trans Angle : Inport  Port=2
  Desired Hip Sag Angle : Inport  Port=3
  Desired Knee Angle : Inport  Port=4
  Desired Ankle Angle : Inport  Port=5
  θ Hip Fron : Inport  Port=6
  θ Hip Trans : Inport  Port=7
  θ Hip Sag : Inport  Port=8
  θ Knee : Inport  Port=9
  θ Ankle : Inport  Port=10
  θ́ HipFron : Inport  Port=11
  θ́ Hip Trans : Inport  Port=12
  θ́ Hip Sag : Inport  Port=13
  θ́ Knee : Inport  Port=14
  θ́ Ankle : Inport  Port=15
  DD Desired Hip Fron Angle : Inport  Port=16
  DD Desired Hip Trans Angle : Inport  Port=17
  DD Desired Hip Sag Angle : Inport  Port=18
  DD Desired Knee Angle : Inport  Port=19
  DD Desired Ankle Angle : Inport  Port=20
  " h͂" : MATLAB Function  TreatAsAtomicUnit=on
  Demux1 : Demux  Outputs=5
  Demux2 : Demux  Outputs=5
  Desired Left Leg Velocity : Subsystem
      mask Display:
      | port_label('output',1,'\theta\prime_d_{ Hip Frontal}','texmode','on');
      | port_label('output',2,'\theta\prime_d_{ Hip Trans}','texmode','on');
      | port_label('output',3,'\theta\prime_d_{ Hip Saggital}','texmode','on');
      | port_label('output',4,'\theta\prime_d_{ Knee}','texmode','on');
      | port_label('output',5,'\theta\prime_d_{ Ankle}','texmode','on');
  Kd1 : Gain  Gain="[5^2  0  0  0  0; 0  5^2  0  0  0; 0  0  5^2  0  0; 0  0  0  5^2  0; 0  0  0  0  5^2]"  Multiplication=Matrix(K*u) (u vector)
  Kd3 : Gain  Gain="[5  0  0  0  0; 0  5  0  0  0; 0  0  5  0  0; 0  0  0  5  0; 0  0  0  0  5]*2"  Multiplication=Matrix(K*u) (u vector)
  Mux{1,4..6} (4 alike) : Mux  Inputs=5
  M͂ : MATLAB Function  TreatAsAtomicUnit=on
  Sum{1,3..5,9} (5 alike) : Sum  Inputs=++|
  Sum2 : Sum
  Sum6 : Sum  Inputs=+-
  Sum7 : Sum
  Sum8 : Sum  Inputs=-+
  Torque Hip Fron : Outport
  Torque Hip Trans : Outport  Port=2
  Torque Hip Sag : Outport  Port=3
  Torque Knee : Outport  Port=4
  Torque Ankle : Outport  Port=5
  wires:
  θ́ Hip Sag/1 -> " h͂"/8(theta_dot_3), Mux6/3
  θ́ Knee/1 -> " h͂"/9(theta_dot_4), Mux6/4
  θ́ Ankle/1 -> " h͂"/10(theta_dot_5), Mux6/5
  θ Hip Sag/1 -> " h͂"/3(theta3), M͂/3(theta3), Mux5/3
  θ Knee/1 -> Mux5/4, " h͂"/4(theta4), M͂/4(theta4)
  θ Ankle/1 -> Mux5/5, M͂/5(theta5), " h͂"/5(theta5)
  " h͂"/1(h_tilda) -> Sum2/2
  M͂/1(M_tilda) -> Sum2/1
  Sum2/1 -> Demux1/1
  DD Desired Hip Sag Angle/1 -> Sum3/1
  DD Desired Knee Angle/1 -> Sum4/1
  DD Desired Ankle Angle/1 -> Sum5/1
  Mux4/1 -> Sum6/1
  Mux5/1 -> Sum6/2
  Sum6/1 -> Kd1/1
  Kd1/1 -> Sum7/1
  Sum7/1 -> Demux2/1
  Mux1/1 -> Sum8/2
  Mux6/1 -> Sum8/1
  Sum8/1 -> Kd3/1
  Sum4/1 -> M͂/9(theta_ddot_4)
  Demux1/5 -> Torque Ankle/1
  Demux1/4 -> Torque Knee/1
  Demux1/3 -> Torque Hip Sag/1
  Demux1/1 -> Torque Hip Fron/1
  Demux1/2 -> Torque Hip Trans/1
  Desired Ankle Angle/1 -> Mux4/5
  Desired Knee Angle/1 -> Mux4/4
  Desired Hip Sag Angle/1 -> Mux4/3
  Desired Hip Fron Angle/1 -> Mux4/1
  Desired Hip Trans Angle/1 -> Mux4/2
  θ Hip Fron/1 -> M͂/1(theta1), " h͂"/1(theta1), Mux5/1
  θ Hip Trans/1 -> " h͂"/2(theta2), M͂/2(theta2), Mux5/2
  θ́ Hip Trans/1 -> " h͂"/7(theta_dot_2), Mux6/2
  θ́ HipFron/1 -> Mux6/1, " h͂"/6(theta_dot_1)
  Desired Left Leg Velocity/1(Left Fron Hip Velocity) -> Mux1/1
  Desired Left Leg Velocity/2(Left Trans Hip Velocity) -> Mux1/2
  Desired Left Leg Velocity/4(Left Knee Velocity) -> Mux1/4
  Demux2/5 -> Sum5/2
  Demux2/4 -> Sum4/2
  Sum5/1 -> M͂/10(theta_ddot_5)
  Demux2/3 -> Sum3/2
  Sum3/1 -> M͂/8(theta_ddot_3)
  Demux2/2 -> Sum1/2
  Sum1/1 -> M͂/7(theta_ddot_2)
  Demux2/1 -> Sum9/2
  Sum9/1 -> M͂/6(theta_ddot_1)
  DD Desired Hip Fron Angle/1 -> Sum9/1
  DD Desired Hip Trans Angle/1 -> Sum1/1
  Desired Left Leg Velocity/3(Left Sag Hip Velocity) -> Mux1/3
  Desired Left Leg Velocity/5(Left Ankle Velocity) -> Mux1/5
  Kd3/1 -> Sum7/2

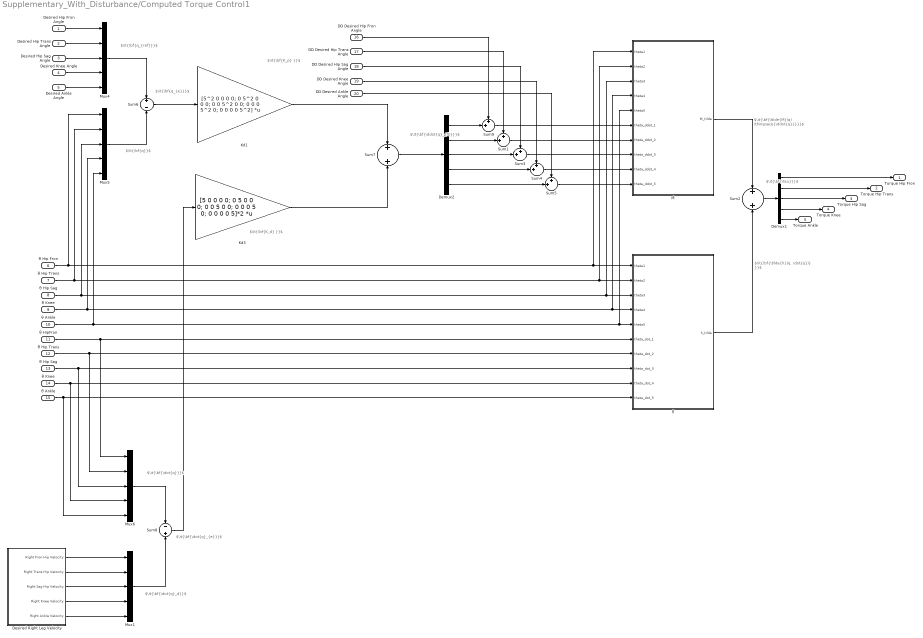
== system Supplementary_With_Disturbance/Computed Torque Control1 ==
  note: $\it{\bf{\ddot{q}_{fb}}}$
  note: $\it{\bf{\dot{q}_{e}}}$
  note: $\it{\bf{K_d} }}$
  note: $\it{\bf{\dot{q}_d}}$
  note: $\it{\bf{\dot{q}}}$
  note: $\it{\bf{K_p} }}$
  note: $\it{\bf{q_{e}}}$
  note: $\it{\bf{\tau}}}$
  note: $\it{\bf{\tilde{h}(q, \dot{q})} }}$
  note: $\it{\bf{q_{ref}}}$
  note: $\it{\bf{q}}$
  note: $\it{\bf{\tilde{M}(q) \thinspace{\ddot{q}}}}}$
  Desired Hip Fron Angle : Inport
  Desired Hip Trans Angle : Inport  Port=2
  Desired Hip Sag Angle : Inport  Port=3
  Desired Knee Angle : Inport  Port=4
  Desired Ankle Angle : Inport  Port=5
  θ Hip Fron : Inport  Port=6
  θ Hip Trans : Inport  Port=7
  θ Hip Sag : Inport  Port=8
  θ Knee : Inport  Port=9
  θ Ankle : Inport  Port=10
  θ́ HipFron : Inport  Port=11
  θ́ Hip Trans : Inport  Port=12
  θ́ Hip Sag : Inport  Port=13
  θ́ Knee : Inport  Port=14
  θ́ Ankle : Inport  Port=15
  DD Desired Hip Fron Angle : Inport  Port=16
  DD Desired Hip Trans Angle : Inport  Port=17
  DD Desired Hip Sag Angle : Inport  Port=18
  DD Desired Knee Angle : Inport  Port=19
  DD Desired Ankle Angle : Inport  Port=20
  " h͂" : MATLAB Function  TreatAsAtomicUnit=on
  Demux1 : Demux  Outputs=5
  Demux2 : Demux  Outputs=5
  Desired Right Leg Velocity : Subsystem
      mask Display:
      | port_label('output',1,'\theta\prime_d_{ Hip Frontal}','texmode','on');
      | port_label('output',2,'\theta\prime_d_{ Hip Trans}','texmode','on');
      | port_label('output',3,'\theta\prime_d_{ Hip Saggital}','texmode','on');
      | port_label('output',4,'\theta\prime_d_{ Knee}','texmode','on');
      | port_label('output',5,'\theta\prime_d_{ Ankle}','texmode','on');
  Kd1 : Gain  Gain="[5^2  0  0  0  0; 0  5^2  0  0  0; 0  0  5^2  0  0; 0  0  0  5^2  0; 0  0  0  0  5^2]"  Multiplication=Matrix(K*u) (u vector)
  Kd3 : Gain  Gain="[5  0  0  0  0; 0  5  0  0  0; 0  0  5  0  0; 0  0  0  5  0; 0  0  0  0  5]*2"  Multiplication=Matrix(K*u) (u vector)
  Mux{1,4..6} (4 alike) : Mux  Inputs=5
  M͂ : MATLAB Function  TreatAsAtomicUnit=on
  Sum{1,3..5,9} (5 alike) : Sum  Inputs=++|
  Sum2 : Sum
  Sum6 : Sum  Inputs=+-
  Sum7 : Sum
  Sum8 : Sum  Inputs=-+
  Torque Hip Fron : Outport
  Torque Hip Trans : Outport  Port=2
  Torque Hip Sag : Outport  Port=3
  Torque Knee : Outport  Port=4
  Torque Ankle : Outport  Port=5
  wires:
  Kd3/1 -> Sum7/2
  DD Desired Hip Trans Angle/1 -> Sum1/1
  DD Desired Hip Fron Angle/1 -> Sum9/1
  Sum9/1 -> M͂/6(theta_ddot_1)
  Demux2/1 -> Sum9/2
  Sum1/1 -> M͂/7(theta_ddot_2)
  Demux2/2 -> Sum1/2
  Sum3/1 -> M͂/8(theta_ddot_3)
  Demux2/3 -> Sum3/2
  Sum5/1 -> M͂/10(theta_ddot_5)
  Demux2/4 -> Sum4/2
  Demux2/5 -> Sum5/2
  Desired Right Leg Velocity/5(Right Ankle Velocity) -> Mux1/5
  Desired Right Leg Velocity/4(Right Knee Velocity) -> Mux1/4
  Desired Right Leg Velocity/3(Right Sag Hip Velocity) -> Mux1/3
  Desired Right Leg Velocity/2(Right Trans Hip Velocity) -> Mux1/2
  Desired Right Leg Velocity/1(Right Fron Hip Velocity) -> Mux1/1
  θ́ HipFron/1 -> " h͂"/6(theta_dot_1), Mux6/1
  θ́ Hip Trans/1 -> Mux6/2, " h͂"/7(theta_dot_2)
  θ Hip Trans/1 -> Mux5/2, M͂/2(theta2), " h͂"/2(theta2)
  θ Hip Fron/1 -> Mux5/1, " h͂"/1(theta1), M͂/1(theta1)
  Desired Hip Trans Angle/1 -> Mux4/2
  Desired Hip Fron Angle/1 -> Mux4/1
  Desired Hip Sag Angle/1 -> Mux4/3
  Desired Knee Angle/1 -> Mux4/4
  Desired Ankle Angle/1 -> Mux4/5
  Demux1/2 -> Torque Hip Trans/1
  Demux1/1 -> Torque Hip Fron/1
  Demux1/3 -> Torque Hip Sag/1
  Demux1/4 -> Torque Knee/1
  Demux1/5 -> Torque Ankle/1
  Sum4/1 -> M͂/9(theta_ddot_4)
  Sum8/1 -> Kd3/1
  Mux6/1 -> Sum8/1
  Mux1/1 -> Sum8/2
  Sum7/1 -> Demux2/1
  Kd1/1 -> Sum7/1
  Sum6/1 -> Kd1/1
  Mux5/1 -> Sum6/2
  Mux4/1 -> Sum6/1
  DD Desired Ankle Angle/1 -> Sum5/1
  DD Desired Knee Angle/1 -> Sum4/1
  DD Desired Hip Sag Angle/1 -> Sum3/1
  Sum2/1 -> Demux1/1
  M͂/1(M_tilda) -> Sum2/1
  " h͂"/1(h_tilda) -> Sum2/2
  θ Ankle/1 -> " h͂"/5(theta5), M͂/5(theta5), Mux5/5
  θ Knee/1 -> M͂/4(theta4), " h͂"/4(theta4), Mux5/4
  θ Hip Sag/1 -> Mux5/3, M͂/3(theta3), " h͂"/3(theta3)
  θ́ Ankle/1 -> Mux6/5, " h͂"/10(theta_dot_5)
  θ́ Knee/1 -> Mux6/4, " h͂"/9(theta_dot_4)
  θ́ Hip Sag/1 -> Mux6/3, " h͂"/8(theta_dot_3)

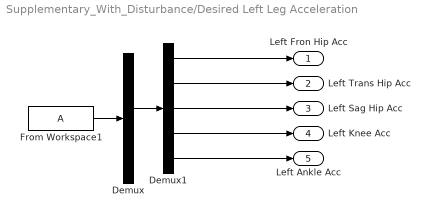
== system Supplementary_With_Disturbance/Desired Left Leg Acceleration ==
  Demux : Demux  Outputs=6
  Demux1 : Demux  Outputs=5
  From Workspace1 : FromWorkspace  VariableName=A
  Left Fron Hip Acc : Outport
  Left Trans Hip Acc : Outport  Port=2
  Left Sag Hip Acc : Outport  Port=3
  Left Knee Acc : Outport  Port=4
  Left Ankle Acc : Outport  Port=5
  wires:
  Demux1/5 -> Left Ankle Acc/1
  Demux1/1 -> Left Fron Hip Acc/1
  Demux1/4 -> Left Knee Acc/1
  Demux1/3 -> Left Sag Hip Acc/1
  Demux1/2 -> Left Trans Hip Acc/1
  From Workspace1/1 -> Demux/1
  Demux/3 -> Demux1/1

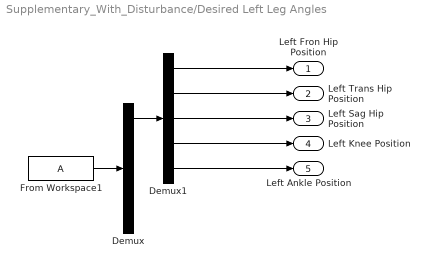
== system Supplementary_With_Disturbance/Desired Left Leg Angles ==
  Demux : Demux  Outputs=6
  Demux1 : Demux  Outputs=5
  From Workspace1 : FromWorkspace  VariableName=A
  Left Fron Hip Position : Outport
  Left Trans Hip Position : Outport  Port=2
  Left Sag Hip Position : Outport  Port=3
  Left Knee Position : Outport  Port=4
  Left Ankle Position : Outport  Port=5
  wires:
  Demux1/5 -> Left Ankle Position/1
  Demux1/1 -> Left Fron Hip Position/1
  Demux1/4 -> Left Knee Position/1
  Demux1/3 -> Left Sag Hip Position/1
  Demux1/2 -> Left Trans Hip Position/1
  From Workspace1/1 -> Demux/1
  Demux/1 -> Demux1/1

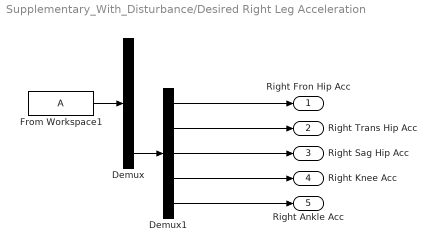
== system Supplementary_With_Disturbance/Desired Right Leg Acceleration ==
  Demux : Demux  Outputs=6
  Demux1 : Demux  Outputs=5
  From Workspace1 : FromWorkspace  VariableName=A
  Right Fron Hip Acc : Outport
  Right Trans Hip Acc : Outport  Port=2
  Right Sag Hip Acc : Outport  Port=3
  Right Knee Acc : Outport  Port=4
  Right Ankle Acc : Outport  Port=5
  wires:
  From Workspace1/1 -> Demux/1
  Demux1/2 -> Right Trans Hip Acc/1
  Demux1/3 -> Right Sag Hip Acc/1
  Demux1/4 -> Right Knee Acc/1
  Demux1/1 -> Right Fron Hip Acc/1
  Demux1/5 -> Right Ankle Acc/1
  Demux/6 -> Demux1/1

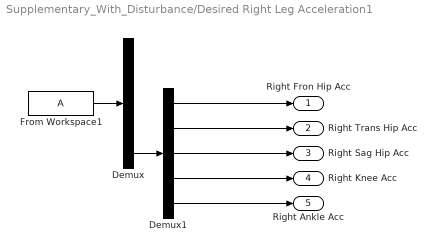
== system Supplementary_With_Disturbance/Desired Right Leg Acceleration1 ==
  Demux : Demux  Outputs=6
  Demux1 : Demux  Outputs=5
  From Workspace1 : FromWorkspace  VariableName=A
  Right Fron Hip Acc : Outport
  Right Trans Hip Acc : Outport  Port=2
  Right Sag Hip Acc : Outport  Port=3
  Right Knee Acc : Outport  Port=4
  Right Ankle Acc : Outport  Port=5
  wires:
  Demux/6 -> Demux1/1
  Demux1/5 -> Right Ankle Acc/1
  Demux1/1 -> Right Fron Hip Acc/1
  Demux1/4 -> Right Knee Acc/1
  Demux1/3 -> Right Sag Hip Acc/1
  Demux1/2 -> Right Trans Hip Acc/1
  From Workspace1/1 -> Demux/1

== system Supplementary_With_Disturbance/Desired Right Leg Angles ==
  Demux : Demux  Outputs=6
  Demux1 : Demux  Outputs=5
  From Workspace1 : FromWorkspace  VariableName=A
  Right Fron Hip Position : Outport
  Right Trans Hip Position : Outport  Port=2
  Right Sag Hip Position : Outport  Port=3
  Right Knee Position : Outport  Port=4
  Right Ankle Position : Outport  Port=5
  wires:
  From Workspace1/1 -> Demux/1
  Demux1/2 -> Right Trans Hip Position/1
  Demux1/3 -> Right Sag Hip Position/1
  Demux1/4 -> Right Knee Position/1
  Demux1/1 -> Right Fron Hip Position/1
  Demux1/5 -> Right Ankle Position/1
  Demux/4 -> Demux1/1

== system Supplementary_With_Disturbance/Desired Right Leg Angles1 ==
  Demux : Demux  Outputs=6
  Demux1 : Demux  Outputs=5
  From Workspace1 : FromWorkspace  VariableName=A
  Right Fron Hip Position : Outport
  Right Trans Hip Position : Outport  Port=2
  Right Sag Hip Position : Outport  Port=3
  Right Knee Position : Outport  Port=4
  Right Ankle Position : Outport  Port=5
  wires:
  Demux/4 -> Demux1/1
  Demux1/5 -> Right Ankle Position/1
  Demux1/1 -> Right Fron Hip Position/1
  Demux1/4 -> Right Knee Position/1
  Demux1/3 -> Right Sag Hip Position/1
  Demux1/2 -> Right Trans Hip Position/1
  From Workspace1/1 -> Demux/1

== system Supplementary_With_Disturbance/I ==
  Mechanism Configuration : sm_lib/Utilities/Mechanism Configuration  UniformGravity=Constant  GravityVector="[0  -9.81 0]"  GravityVectorUnits=m/s^2  GravityUnits=m/s^2  LinearizationDelta=0.001  JointModeTransitionNonlinearIterations=2
  Solver Configuration : nesl_utility/Solver Configuration  PhysicalDomain=network_engine_domain  SubClassName=solver  LeftPortType=input  RightPortType=generic  Tones=[]  Harmonics=[]  SimulateNoise=off  Profile=off  UseLocalSampling=off  EnableSwitchedLinearOptims=on  FrequencyDomain=off  UseCCode=off  RelTol=0.001  AbsTol=1e-06  MinStep=1e-09  ToWorkspace=off  RevertToSquareIcSolve=off  NumHomotopyIterations=100  PhasorMode=off  PhasorModeNumHarmonics=1  DoDC=on  ResidualTolerance=0.1  UseLocalSolver=off  LocalSolverChoice=NE_BACKWARD_EULER_ADVANCER  LocalSolverSampleTime=0.001  DoFixedCost=off  MaxNonlinIter=3  MaxModeIter=2  ComputeImpulses=off  ImpulseIterations=2  LinearAlgebra=Sparse  EquationFormulation=NE_TIME_EF  DelaysMemoryBudget=1024  AutomaticFiltering=on  FilteringTimeConstant=0.001  PartitionStorageMethod=AS_NEEDED  PartitionMemoryBudget=1024  PartitionMethod=FAST
  World Frame : sm_lib/Frames and Transforms/World Frame
  I : PMIOPort  Side=Right
  connections:
  Solver Configuration/RConn1 -- I/RConn1 -- Mechanism Configuration/RConn1 -- World Frame/RConn1
